simulink model "feedback_linearization_PD"  (R2015a)
settings: Solver=ode4  StartTime=0.0  StopTime=tsim  FixedStep=0.01  MaxStep=0.01  RelTol=1e-3
settings Model: Creator=peixeboi  LastModifiedBy=peixeboi
settings SolverCC: ZeroCrossControl=DisableAll

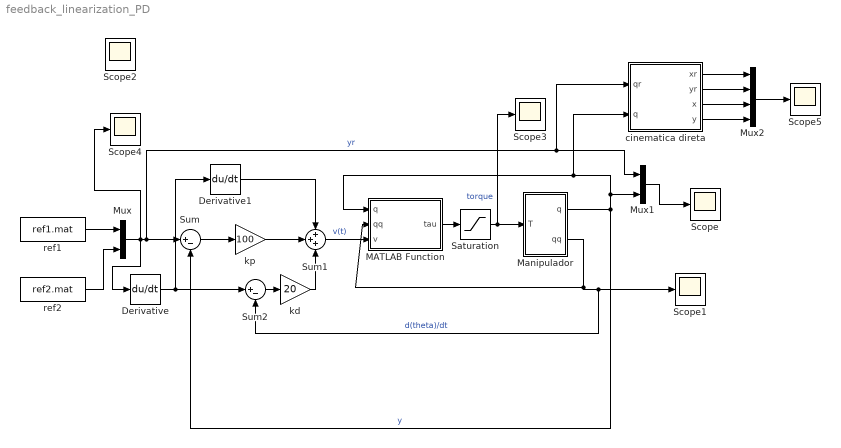
== system feedback_linearization_PD ==
  Derivative : Derivative
  Derivative1 : Derivative
  MATLAB Function : MATLAB Function  TreatAsAtomicUnit=on
  Manipulador : Subsystem
  Mux : Mux  Inputs=2
  Mux1 : Mux  Inputs=2
  Mux2 : Mux
  Saturation : Saturate  UpperLimit=100  LowerLimit=-100
  Scope{,1..5} (6 alike) : Scope
      Scope settings: ShowLegends=on  SaveName=x
      Scope1 settings: ShowLegends=on
      Scope3 settings: ShowLegends=on  SaveName=ScopeData3
      Scope4 settings: ShowLegends=on  SaveName=ScopeData4
      Scope5 settings: ShowLegends=on  SaveName=xy
      Scope2 settings: SaveName=ScopeData2
  Sum : Sum  Inputs=|+-
  Sum1 : Sum  Inputs=+++
  Sum2 : Sum  Inputs=|+-
  cinematica direta : MATLAB Function  TreatAsAtomicUnit=on
  kd : Gain  Gain=20
  kp : Gain  Gain=100
  ref1 : FromFile  FileName=ref1.mat  SampleTime=0
  ref2 : FromFile  FileName=ref2.mat  SampleTime=0
  wires:
  Manipulador/2(qq) -> MATLAB Function/2(qq), Sum2/2, Scope1/1  "d(theta)/dt"
  Manipulador/1(q) -> Mux1/2, cinematica direta/2(q), MATLAB Function/1(q), Sum/2  "y"
  ref1/1 -> Mux/1
  ref2/1 -> Mux/2
  Sum/1 -> kp/1
  Mux/1 -> Scope4/1, Derivative/1, cinematica direta/1(qr), Mux1/1, Sum/1  "yr"
  Derivative/1 -> Derivative1/1, Sum2/1
  Sum2/1 -> kd/1
  kp/1 -> Sum1/2
  kd/1 -> Sum1/3
  Derivative1/1 -> Sum1/1
  Sum1/1 -> MATLAB Function/3(v)  "v(t)"
  MATLAB Function/1(tau) -> Saturation/1
  Mux1/1 -> Scope/1
  Saturation/1 -> Scope3/1, Manipulador/1(T)  "torque"
  Mux2/1 -> Scope5/1
  cinematica direta/1(xr) -> Mux2/1
  cinematica direta/2(yr) -> Mux2/2
  cinematica direta/3(x) -> Mux2/3
  cinematica direta/4(y) -> Mux2/4

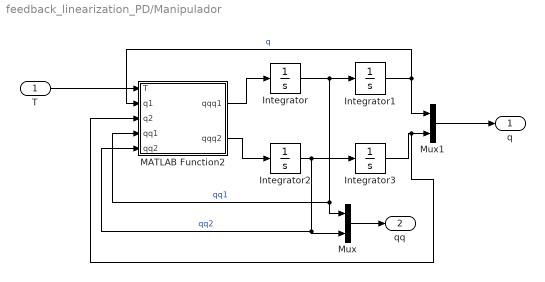
== system feedback_linearization_PD/Manipulador ==
  T : Inport
  Integrator : Integrator
  Integrator1 : Integrator
  Integrator2 : Integrator
  Integrator3 : Integrator  InitialCondition=pi/4
  MATLAB Function2 : MATLAB Function  TreatAsAtomicUnit=on
  Mux : Mux  Inputs=2
  Mux1 : Mux  Inputs=2
  q : Outport  PortDimensions=2
  qq : Outport  Port=2  PortDimensions=2
  wires:
  Integrator/1 -> MATLAB Function2/4(qq1), Mux/1, Integrator1/1  "qq1"
  T/1 -> MATLAB Function2/1(T)
  MATLAB Function2/1(qqq1) -> Integrator/1
  MATLAB Function2/2(qqq2) -> Integrator2/1
  Integrator2/1 -> MATLAB Function2/5(qq2), Mux/2, Integrator3/1  "qq2"
  Mux/1 -> qq/1
  Integrator1/1 -> Mux1/1, MATLAB Function2/2(q1)  "q"
  Integrator3/1 -> MATLAB Function2/3(q2), Mux1/2
  Mux1/1 -> q/1

== matlab function feedback_linearization_PD/cinematica direta ==
  data: qr input; xr output; yr output; q input; x output; y output
function [xr, yr, x, y] = cin_dir(qr, q)
L1 = 0.6;
L2 = 0.6;

x = L1*cos(q(1))+L2*cos(q(1)+q(2));
y = L1*sin(q(1))+L2*sin(q(1)+q(2));

xr = L1*cos(qr(1))+L2*cos(qr(1)+qr(2));
yr = L1*sin(qr(1))+L2*sin(qr(1)+qr(2));

== matlab function feedback_linearization_PD/MATLAB Function ==
  data: q input; tau output; qq input; v input
function tau = fcn(q, qq, v)
q1=q(1);
q2=q(2);
qq1=qq(1);
qq2=qq(2);
m1 = 2.2;
m2 = 2.2;
L1 = 0.6;
L2 = 0.6;
g=9.81;
l1 = 0.3;
l2 = 0.3;
I1 = 0.066;
I2 = 0.066;
mp=4;

H = zeros(2,1);
H(1) = -L1*(m2*l2+mp*L2)*sin(q2)*(2*qq1*qq2+qq2^2)+(m1*l1+(m2+mp)*L1)*g*cos(q1)+(m2*l2+mp*L1)*g*cos(q1+q2);
H(2) = L1*(m2*l2+mp*L2)*sin(q2)*qq1^2+(m2*l2+mp*L1)*g*cos(q1+q2);

M = zeros(2,2);
M(1,1) = I1+I2+m1*l1^2+(m2+mp)*L1^2+m2*(l2^2+L2^2)+2*L1*(m2*l2+mp*L2)*cos(q2);
M(1,2) = I2+m2*l2^2+mp*L2^2+L1*(m2*l2+mp*L2)*cos(q2);
M(2,1) = M(1,2);
M(2,2) = I2+m2*l2^2+mp*L2^2;

tau = M*v+H;

== matlab function feedback_linearization_PD/Manipulador/MATLAB Function2 ==
  data: T input; q1 input; q2 input; qqq1 output; qq1 input; qq2 input; qqq2 output
function [qqq1, qqq2] = Manip(T, q1, q2, qq1, qq2)
m1 = 2.2;
m2 = 2.2;
L1 = 0.6;
L2 = 0.6;
g=9.81;
l1 = 0.3;
l2 = 0.3;
I1 = 0.066;
I2 = 0.066;
mp=4;

H = zeros(2,1);
H(1) = -L1*(m2*l2+mp*L2)*sin(q2)*(2*qq1*qq2+qq2^2)+(m1*l1+(m2+mp)*L1)*g*cos(q1)+(m2*l2+mp*L1)*g*cos(q1+q2);
H(2) = L1*(m2*l2+mp*L2)*sin(q2)*qq1^2+(m2*l2+mp*L1)*g*cos(q1+q2);

M = zeros(2,2);
M(1,1) = I1+I2+m1*l1^2+(m2+mp)*L1^2+m2*(l2^2+L2^2)+2*L1*(m2*l2+mp*L2)*cos(q2);
M(1,2) = I2+m2*l2^2+mp*L2^2+L1*(m2*l2+mp*L2)*cos(q2);
M(2,1) = M(1,2);
M(2,2) = I2+m2*l2^2+mp*L2^2;

B = [5*qq1;
    5*qq2];

b = T - H - B; 
qqq = M\b;
qqq1 = qqq(1);
qqq2 = qqq(2);
end
